simulink model "three_phase_induction_motor"  (R2023b)
settings: Solver=VariableStepAuto  StartTime=0.0  StopTime=10.0  RelTol=1e-3
libraries: spsACVoltageSourceLib x3, spsAsynchronousMachinepuUnitsLib x1, spsGroundLib x1, sps_lib x1
settings Model: Creator=dhana  LastModifiedBy=dhana

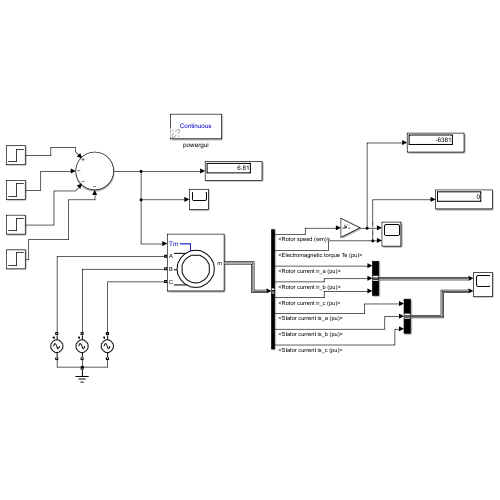
[thumbnail: Simulink's stored preview of the top-level diagram]
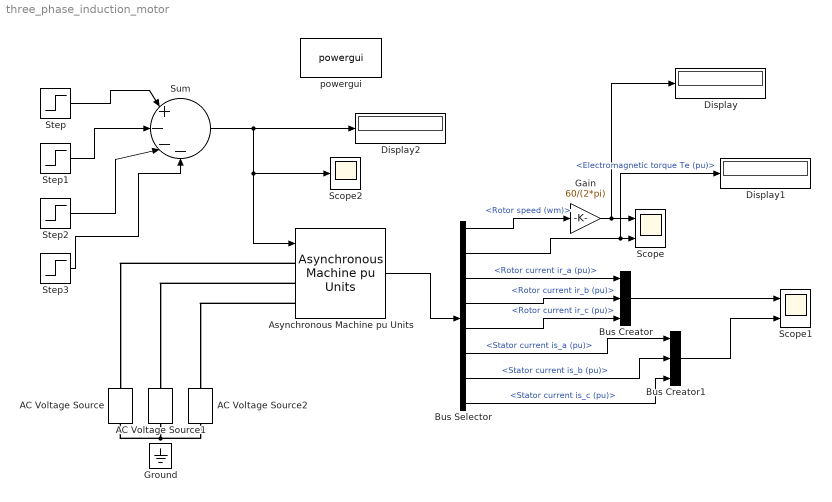
== system three_phase_induction_motor ==
  AC Voltage Source : spsACVoltageSourceLib/AC Voltage Source  Amplitude=326.54  Phase=0  Frequency=50  SampleTime=0  Measurements=None  BusType=swing  Pref=10e3  Qref=0  Qmin=-inf  Qmax=+inf
  AC Voltage Source1 : spsACVoltageSourceLib/AC Voltage Source  Amplitude=326.54  Phase=0  Frequency=50  SampleTime=0  Measurements=None  BusType=swing  Pref=10e3  Qref=0  Qmin=-inf  Qmax=+inf
  AC Voltage Source2 : spsACVoltageSourceLib/AC Voltage Source  Amplitude=326.54  Phase=0  Frequency=50  SampleTime=0  Measurements=None  BusType=swing  Pref=10e3  Qref=0  Qmin=-inf  Qmax=+inf
  Asynchronous Machine pu Units : spsAsynchronousMachinepuUnitsLib/Asynchronous Machine pu Units  RotorType=Squirrel-cage  PresetModel="15:  5.4 HP (4KW)   400 V  50Hz 1430 RPM"  MechanicalLoad=Torque Tm  ShowDetailedParameters=on  ReferenceFrame=Rotor  Units=pu  MeasurementBus=off  NominalParameters=[4000 400 50]  VoltageRatio=1  Stator=[0.03513 0.04586]  Rotor=[0.03488 0.04586]  Cage1=[0.01909 0.0397]  Cage2=[0.01909 0.0397]  Lm=1.352  Mechanical=[0.0404 0.01841 2]  PolePairs=2  InitialConditions="[ 1,0   0,0,0   0,0,0 ]"  SimulateSaturation=off  Saturation="[0.212,0.4201,0.8125,1.0979,1.4799,2.2457,3.2586,4.5763,6.4763 ;   0.5,0.7,0.9,1,1.1,1.2 ,1.3,1.4,1.5]"  LoadFlowParameters=0  TsPowergui=0  TsBlock=-1  IterativeModel=Trapezoidal non iterative  IterativeDiscreteModel=Trapezoidal non iterative  Pmec=0
      settings: LibrarySourceBlock=|
      | sps_lib/Electrical Machines/Asynchronous Machine
      | pu Units
  Bus Creator : BusCreator  Inputs=3
  Bus Creator1 : BusCreator  Inputs=3
  Bus Selector : BusSelector  OutputSignals=Mechanical.Rotor speed (wm),Mechanical.Electromagnetic torque Te (pu),Rotor measurements.Rotor current ir_a (pu),Rotor measurements.Rotor current ir_b (pu),Rotor measurements.Rotor current ir_c (pu),Stator measurements.Stator current is_a (pu),Stator measurements.Stator current is_b (pu),Stator measurements.Stator current is_c (pu)
  Display : Display
  Display1 : Display
  Display2 : Display
  Gain : Gain  Gain=60/(2*pi)
  Ground : spsGroundLib/Ground  LConnTagsString=a
  Scope : Scope  NumInputPorts=2
  Scope1 : Scope  NumInputPorts=2
  Scope2 : Scope
  Step : Step  Time=3  After=26.72  SampleTime=0
  Step1 : Step  Time=5  After=13.23  SampleTime=0
  Step2 : Step  Time=10  After=6.68  SampleTime=0
  Step3 : Step  Time=13  After=6.68  SampleTime=0
  Sum : Sum  Inputs=|+---
  powergui : sps_lib/powergui  Priority=1  SimulationMode=Continuous  SampleTime=50e-6  frequency=60  Iterations=50  frequencyindice=50  Pbase=100e6  ErrMax=1e-4  UnitsV=kV  UnitsW=MW  buscounter=0  FunctionMessages=off  echomessages=off  EnableUseOfTLC=off  CurrentSourceSwitches=off  DisableSnubberDevices=off  DisableRonSwitches=off  DisableVfSwitches=off  DisplayEquations=off  AutomaticDiscreteSolvers=off  SolverType=Tustin/Backward Euler (TBE)  Interpol=off  ExternalGateDelay=off  methode=off  Ts=100  x0status=blocks  SPID=on  SwTol=0  HookPort=off  NonlinearTolerance=1e-4  nMaxIteration=100  ContinueOnMaxIteration=off  RestoreLinks=warning  ResistiveCurrentMeasurement=off  Frange=[0:2:500]  Ylog=off  Xlog=on  ShowGrid=off  save=off  variable=ZData  structure=0  ZoomFFT=off  StartTime=0.0  cycles=1  DisplayStyle=1  fundamental=60  FreqAxis=off  MaxFrequency=1000  frequencyindicesteady=1  RmsSteady=1  display=off
  wires:
  Asynchronous Machine pu Units/1 -> Bus Selector/1
  Bus Creator/1 -> Scope1/1
  Bus Creator1/1 -> Scope1/2
  Gain/1 -> Display/1, Scope/1
  Step/1 -> Sum/1
  Step1/1 -> Sum/2
  Step2/1 -> Sum/3
  Step3/1 -> Sum/4
  Sum/1 -> Scope2/1, Asynchronous Machine pu Units/1, Display2/1
  Bus Selector/1 -> Gain/1  "<Rotor speed (wm)>"
  Bus Selector/2 -> Display1/1, Scope/2  "<Electromagnetic torque Te (pu)>"
  Bus Selector/3 -> Bus Creator/1  "<Rotor current ir_a (pu)>"
  Bus Selector/4 -> Bus Creator/2  "<Rotor current ir_b (pu)>"
  Bus Selector/5 -> Bus Creator/3  "<Rotor current ir_c (pu)>"
  Bus Selector/6 -> Bus Creator1/1  "<Stator current is_a (pu)>"
  Bus Selector/7 -> Bus Creator1/2  "<Stator current is_b (pu)>"
  Bus Selector/8 -> Bus Creator1/3  "<Stator current is_c (pu)>"
  connections:
  Asynchronous Machine pu Units/LConn1 -- AC Voltage Source/RConn1
  Asynchronous Machine pu Units/LConn2 -- AC Voltage Source1/RConn1
  Asynchronous Machine pu Units/LConn3 -- AC Voltage Source2/RConn1
  AC Voltage Source2/LConn1 -- AC Voltage Source1/LConn1 -- AC Voltage Source/LConn1
